simulink model "lab1"  (R2024a)
settings: Solver=ode45  StartTime=0.0  StopTime=10.0  MaxStep=1/360  RelTol=1e-3
undefined symbols (not defined in the file): b, k, m
settings Model: Creator=Kamil Kowalczyk  LastModifiedBy=Kamil Kowalczyk

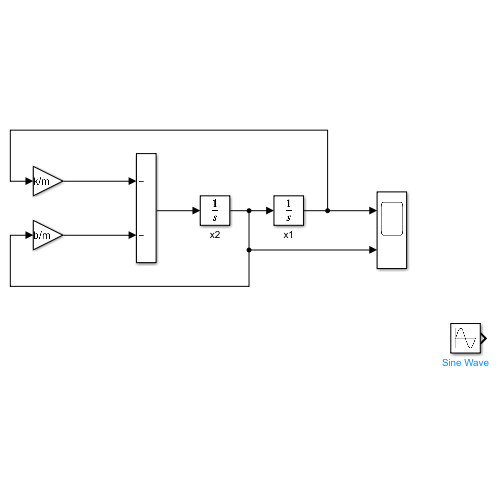
[thumbnail: Simulink's stored preview of the top-level diagram]
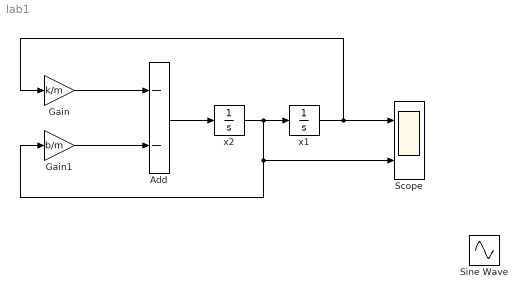
== system lab1 ==
  Add : Sum  Inputs=--
  Gain : Gain  Gain=k/m
  Gain1 : Gain  Gain=b/m
  Scope : Scope  NumInputPorts=2
  Sine Wave : Sin  Frequency=2*pi*1  SampleTime=0
  x1 : Integrator  InitialCondition=1
  x2 : Integrator
  wires:
  x2/1 -> Gain1/1, Scope/2, x1/1
  Gain/1 -> Add/1
  x1/1 -> Gain/1, Scope/1
  Add/1 -> x2/1
  Gain1/1 -> Add/2
